simulink model "lec1_pg16"  (R2024b)
settings: Solver=VariableStepAuto  StartTime=0.0  StopTime=100.0  RelTol=1e-3
settings Model: Creator=ramse  LastModifiedBy=ramse

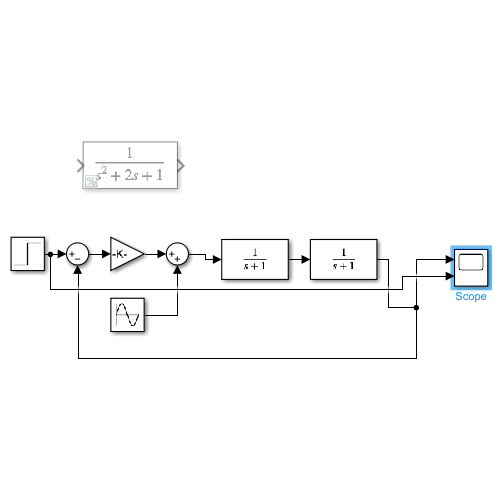
[thumbnail: Simulink's stored preview of the top-level diagram]
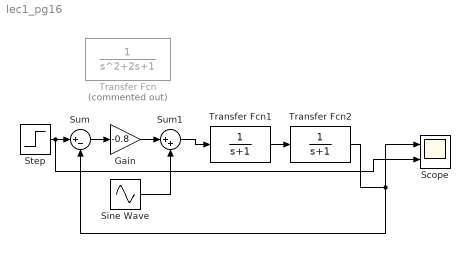
== system lec1_pg16 ==
  Gain : Gain  Gain=-0.8
  Scope : Scope  NumInputPorts=2
  Sine Wave : Sin  SampleTime=0
  Step : Step  SampleTime=0
  Sum : Sum  Inputs=|+-
  Sum1 : Sum  Inputs=|++
  Transfer Fcn : TransferFcn  Commented=on  Denominator=[1, 2, 1]
  Transfer Fcn1 : TransferFcn  Denominator=[1 1]
  Transfer Fcn2 : TransferFcn  Denominator=[1 1]
  wires:
  Step/1 -> Sum/1, Scope/2
  Gain/1 -> Sum1/1
  Sum/1 -> Gain/1
  Sine Wave/1 -> Sum1/2
  Sum1/1 -> Transfer Fcn1/1
  Transfer Fcn1/1 -> Transfer Fcn2/1
  Transfer Fcn2/1 -> Scope/1, Sum/2
